simulink model "SerialComm"  (R2021a)
settings: Solver=FixedStepAuto  StartTime=0.0  StopTime=10.0  FixedStep=1e-3  RelTol=1e-3  EnableMultiTasking=on
undefined symbols (not defined in the file): A0, A1, D0, D1, D10, D11, D12, D13, D2, D3, D4, D5, D6, D7, D8, D9, magnitude, PTA0, PTA1, PTA2, PTB2, PTB23, PTB3, PTB9, PTC16, PTC17, PTC2, PTC3, PTC4, PTD0, PTD1, PTD2, PTD3
libraries: frdmk64flib x23, etargetslib x6, dspstat3 x1, simulink x1
(part 1 of 3)
settings Model: ExtModeTrigDuration=5  Creator=Arun Mistry  LastModifiedBy=Arun Mistry
settings OptimizationCC: EnhancedBackFolding=on  PassReuseOutputArgsAs=Individual arguments  ZeroExternalMemoryAtStartup=off  ZeroInternalMemoryAtStartup=off  MaxStackSize=64  OptimizeBlockOrder=speed  DifferentSizesBufferReuse=on  OptimizationCustomize=off  EfficientTunableParamExpr=on
settings DebuggingCC: ParameterTunabilityLossMsg=error
settings HardwareCC: ProdBitPerPointer=32  ProdBitPerSizeT=32  ProdBitPerPtrDiffT=32  ProdLargestAtomicInteger=Long  ProdLargestAtomicFloat=Double  ProdWordSize=32  ProdHWDeviceType=ARM Compatible->ARM Cortex
settings SFSimCC: MATLABDynamicMemAlloc=off
settings RTWCC: SystemTargetFile=ert.tlc  HardwareBoard=NXP FRDM-K64F  TLCOptions="-aInlineSetEventsForThisBaseRateFcn=TLC_FALSE -aSuppressMultiTaskScheduler=TLC_FALSE  -aRateBasedStepFcn=0"  TemplateMakefile=ert_default_tmf  Toolchain=GNU Tools for ARM Embedded Processors
settings CodeAppCC: ForceParamTrailComments=on  IgnoreCustomStorageClasses=off  OperatorAnnotations=on  SimulinkDataObjDesc=on  SFDataObjDesc=on  InsertBlockDesc=on
settings ERTTargetCC: ExtModeTransport=4  ExtModeMexFile=sendToCommService

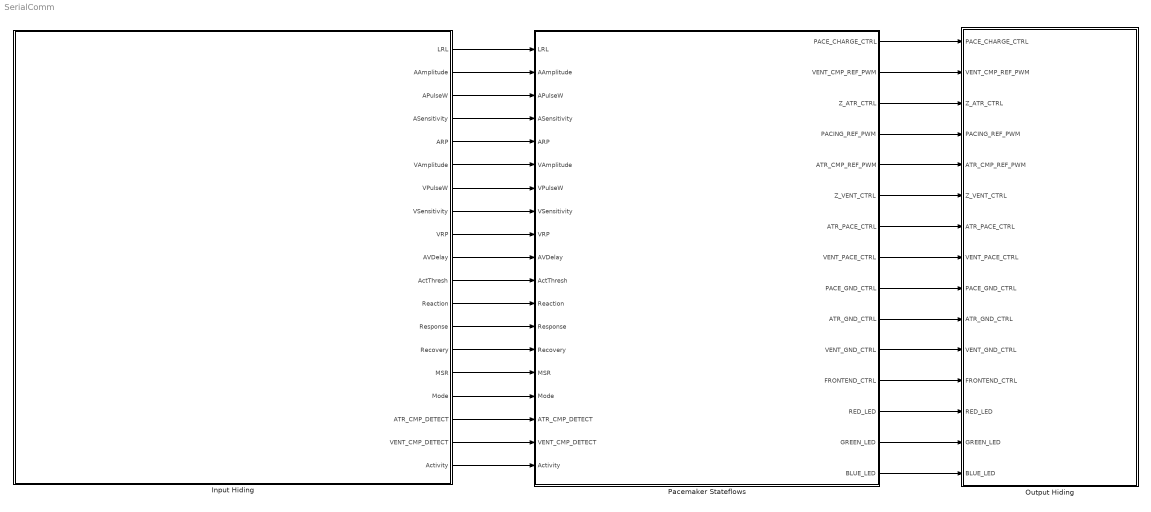
== system SerialComm ==
  Input Hiding : Subsystem
  Output Hiding : Subsystem
  Pacemaker Stateflows : Stateflow chart  TreatAsAtomicUnit=on
      settings: PortSchema="{\"entries\":[{\"content\":{\"sides\":[{\"content\":{\"connectorIds\":[\"In1\",\"In2\",\"In3\",\"In4\",\"In5\",\"In6\",\"In7\",\"In8\",\"In9\",\"In17\",\"In11\",\"In10\",\"In12\",\"In14\",\"In19\",\"In13\",\"In15\",\"In16\",\"In18\"]},\"type\":\"ConnectorPlacement.EquallySpacedRectSide\",\"uuid\":\"6f24296b-9994-4871-8227-e053a3629335\"},{\"content\":{\"connectorIds\":[\"Out1\",\"Out2\",\"Out3\",\"Out4\",\"Out5\",\"Out6\",\"Out7\",\"Out8\",\"Out9\",\"Out10\",\"Out11\",\"Out12\",\"Out13\",\"Out14\",\"Out15\"],\"side\":\"RIGHT\"},\"type\":\"ConnectorPlacement.EquallySpacedRectSide\",\"uuid\":\"36cf1f29-c3ea-48aa-b003-da737efff16a\"},{\"content\":{\"connectorIds\":[],\"side\":\"TOP\"},\"type\":\"ConnectorPlacement.EquallySpacedRectSide\",\"uuid\":\"8330eb51-0bc3-4d96-96ed-331fbb159cdb\"}]},\"type\":\"ConnectorPlacement.EquallySpacedConnector\",\"uuid\":\"1e79ed8a-065e-4a3c-97dd-23eb49490e0b\"}],\"packageUris\":[\"http://schema.mathworks.com/mf0/Connector/R2020b\"],\"version\":\"1.0\"}"
  wires:
  Input Hiding/14(Recovery) -> Pacemaker Stateflows/14(Recovery)
  Input Hiding/16(Mode) -> Pacemaker Stateflows/13(Mode)
  Pacemaker Stateflows/9(PACE_GND_CTRL) -> Output Hiding/9(PACE_GND_CTRL)
  Input Hiding/11(ActThresh) -> Pacemaker Stateflows/11(ActThresh)
  Input Hiding/9(VRP) -> Pacemaker Stateflows/9(VRP)
  Pacemaker Stateflows/5(ATR_CMP_REF_PWM) -> Output Hiding/5(ATR_CMP_REF_PWM)
  Input Hiding/8(VSensitivity) -> Pacemaker Stateflows/8(VSensitivity)
  Input Hiding/13(Response) -> Pacemaker Stateflows/12(Response)
  Input Hiding/19(Activity) -> Pacemaker Stateflows/18(Activity)
  Input Hiding/6(VAmplitude) -> Pacemaker Stateflows/6(VAmplitude)
  Pacemaker Stateflows/2(VENT_CMP_REF_PWM) -> Output Hiding/2(VENT_CMP_REF_PWM)
  Pacemaker Stateflows/8(VENT_PACE_CTRL) -> Output Hiding/8(VENT_PACE_CTRL)
  Pacemaker Stateflows/12(FRONTEND_CTRL) -> Output Hiding/12(FRONTEND_CTRL)
  Input Hiding/10(AVDelay) -> Pacemaker Stateflows/17(AVDelay)
  Pacemaker Stateflows/13(RED_LED) -> Output Hiding/13(RED_LED)
  Pacemaker Stateflows/3(Z_ATR_CTRL) -> Output Hiding/3(Z_ATR_CTRL)
  Pacemaker Stateflows/14(GREEN_LED) -> Output Hiding/14(GREEN_LED)
  Input Hiding/15(MSR) -> Pacemaker Stateflows/19(MSR)
  Input Hiding/4(ASensitivity) -> Pacemaker Stateflows/4(ASensitivity)
  Input Hiding/1(LRL) -> Pacemaker Stateflows/1(LRL)
  Input Hiding/5(ARP) -> Pacemaker Stateflows/5(ARP)
  Pacemaker Stateflows/11(VENT_GND_CTRL) -> Output Hiding/11(VENT_GND_CTRL)
  Input Hiding/12(Reaction) -> Pacemaker Stateflows/10(Reaction)
  Input Hiding/2(AAmplitude) -> Pacemaker Stateflows/2(AAmplitude)
  Pacemaker Stateflows/1(PACE_CHARGE_CTRL) -> Output Hiding/1(PACE_CHARGE_CTRL)
  Input Hiding/3(APulseW) -> Pacemaker Stateflows/3(APulseW)
  Pacemaker Stateflows/4(PACING_REF_PWM) -> Output Hiding/4(PACING_REF_PWM)
  Input Hiding/18(VENT_CMP_DETECT) -> Pacemaker Stateflows/16(VENT_CMP_DETECT)
  Input Hiding/17(ATR_CMP_DETECT) -> Pacemaker Stateflows/15(ATR_CMP_DETECT)
  Pacemaker Stateflows/7(ATR_PACE_CTRL) -> Output Hiding/7(ATR_PACE_CTRL)
  Input Hiding/7(VPulseW) -> Pacemaker Stateflows/7(VPulseW)
  Pacemaker Stateflows/10(ATR_GND_CTRL) -> Output Hiding/10(ATR_GND_CTRL)
  Pacemaker Stateflows/6(Z_VENT_CTRL) -> Output Hiding/6(Z_VENT_CTRL)
  Pacemaker Stateflows/15(BLUE_LED) -> Output Hiding/15(BLUE_LED)

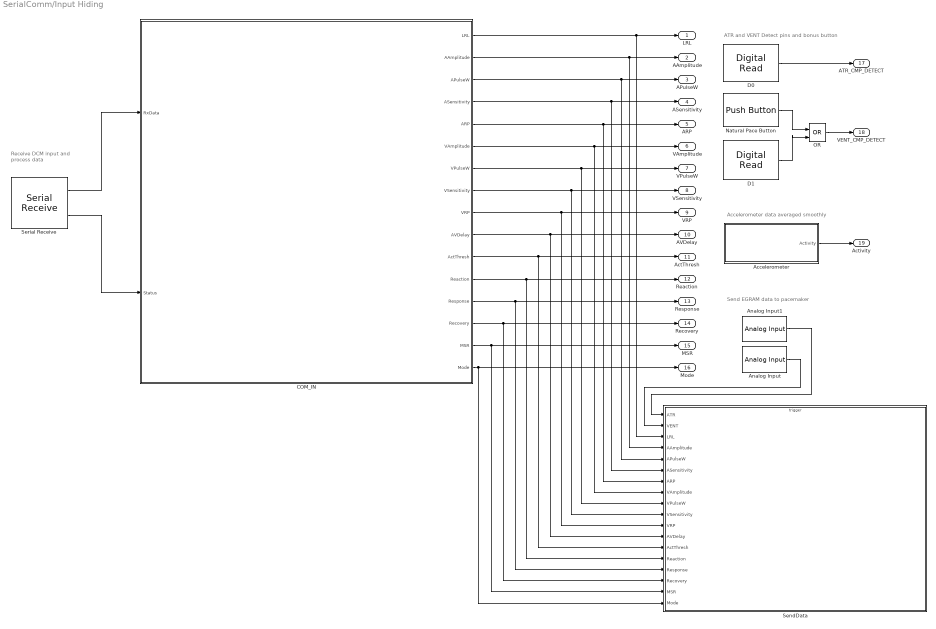
== system SerialComm/Input Hiding ==
  note: ATR and VENT Detect pins and bonus button
  note: Accelerometer data averaged smoothly
  note: Send EGRAM data to pacemaker
  note: Receive DCM input
      | and process data
  Accelerometer : Subsystem
  Analog Input : frdmk64flib/Analog Input  Whichpin=PTB3 (A1)  SampleTime=-1
  Analog Input1 : frdmk64flib/Analog Input  Whichpin=PTB2 (A0)  SampleTime=-1
  COM_IN : Stateflow chart  TreatAsAtomicUnit=on
  D0 : frdmk64flib/Digital Read  Whichpin=PTC16 (D0)  SampleTime=-1
  D1 : frdmk64flib/Digital Read  Whichpin=PTC17 (D1)  SampleTime=-1
  Natural Pace Button : frdmk64flib/Push Button  Whichswitch=SW3  SampleTime1=-1
  OR : Logic  Operator=OR  IconShape=distinctive  AllPortsSameDT=off  OutDataTypeStr=boolean
  SendData : Subsystem  TreatAsAtomicUnit=on
  Serial Receive : frdmk64flib/Serial Receive  SCIModule=0  Baudrate=uint32(9600)  Parity=None  StopBits=1  HardwareFlowControl=None  ByteOrder=LittleEndian  DataType=uint8  DataLength=22  BlockingMode=off  OutputStatus=on  SampleTime=-1
  LRL : Outport  OutDataTypeStr=uint16
  AAmplitude : Outport  Port=2  OutDataTypeStr=uint8
  APulseW : Outport  Port=3  OutDataTypeStr=uint8
  ASensitivity : Outport  Port=4  OutDataTypeStr=uint8
  ARP : Outport  Port=5  OutDataTypeStr=uint16
  VAmplitude : Outport  Port=6  OutDataTypeStr=uint8
  VPulseW : Outport  Port=7  OutDataTypeStr=uint8
  VSensitivity : Outport  Port=8  OutDataTypeStr=uint8
  VRP : Outport  Port=9  OutDataTypeStr=uint16
  AVDelay : Outport  Port=10  OutDataTypeStr=uint16
  ActThresh : Outport  Port=11  OutDataTypeStr=double
  Reaction : Outport  Port=12  OutDataTypeStr=uint8
  Response : Outport  Port=13  OutDataTypeStr=uint8
  Recovery : Outport  Port=14  OutDataTypeStr=uint16
  MSR : Outport  Port=15  OutDataTypeStr=uint16
  Mode : Outport  Port=16  OutDataTypeStr=uint8
  ATR_CMP_DETECT : Outport  Port=17  OutDataTypeStr=boolean
  VENT_CMP_DETECT : Outport  Port=18  OutDataTypeStr=boolean
  Activity : Outport  Port=19  OutDataTypeStr=double
  wires:
  COM_IN/3(APulseW) -> APulseW/1, SendData/5(APulseW)
  COM_IN/7(VPulseW) -> VPulseW/1, SendData/9(VPulseW)
  COM_IN/9(VRP) -> VRP/1, SendData/11(VRP)
  COM_IN/5(ARP) -> ARP/1, SendData/7(ARP)
  D0/1 -> ATR_CMP_DETECT/1
  COM_IN/1(LRL) -> LRL/1, SendData/3(LRL)
  COM_IN/10(AVDelay) -> AVDelay/1, SendData/12(AVDelay)
  COM_IN/6(VAmplitude) -> VAmplitude/1, SendData/8(VAmplitude)
  COM_IN/2(AAmplitude) -> AAmplitude/1, SendData/4(AAmplitude)
  Accelerometer/1(Activity) -> Activity/1
  COM_IN/12(Reaction) -> Reaction/1, SendData/14(Reaction)
  COM_IN/13(Response) -> Response/1, SendData/15(Response)
  COM_IN/14(Recovery) -> Recovery/1, SendData/16(Recovery)
  COM_IN/15(MSR) -> MSR/1, SendData/17(MSR)
  COM_IN/11(ActThresh) -> ActThresh/1, SendData/13(ActThresh)
  D1/1 -> OR/2
  OR/1 -> VENT_CMP_DETECT/1
  Natural Pace Button/1 -> OR/1
  COM_IN/4(ASensitivity) -> ASensitivity/1, SendData/6(ASensitivity)
  COM_IN/8(VSensitivity) -> VSensitivity/1, SendData/10(VSensitivity)
  Serial Receive/2 -> COM_IN/2(Status)
  Serial Receive/1 -> COM_IN/1(RxData)
  COM_IN/16(Mode) -> Mode/1, SendData/18(Mode)
  Analog Input/1 -> SendData/2(VENT)
  Analog Input1/1 -> SendData/1(ATR)

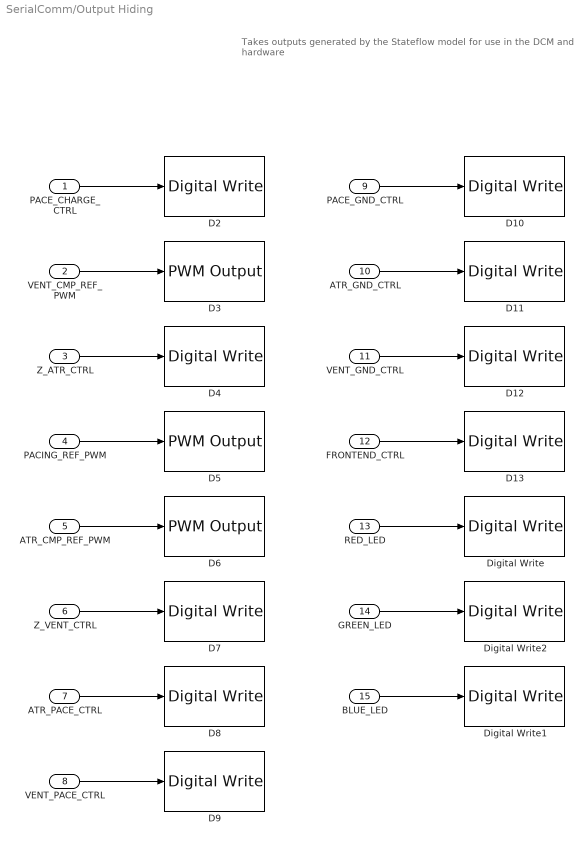
== system SerialComm/Output Hiding ==
  note: Takes outputs generated by the Stateflow model for use in the DCM and hardware
  PACE_CHARGE_CTRL : Inport  OutDataTypeStr=boolean
  VENT_CMP_REF_PWM : Inport  Port=2  OutDataTypeStr=uint8
  Z_ATR_CTRL : Inport  Port=3  OutDataTypeStr=boolean
  PACING_REF_PWM : Inport  Port=4  OutDataTypeStr=uint8
  ATR_CMP_REF_PWM : Inport  Port=5  OutDataTypeStr=uint8
  Z_VENT_CTRL : Inport  Port=6  OutDataTypeStr=boolean
  ATR_PACE_CTRL : Inport  Port=7  OutDataTypeStr=boolean
  VENT_PACE_CTRL : Inport  Port=8  OutDataTypeStr=boolean
  PACE_GND_CTRL : Inport  Port=9  OutDataTypeStr=boolean
  ATR_GND_CTRL : Inport  Port=10  OutDataTypeStr=boolean
  VENT_GND_CTRL : Inport  Port=11  OutDataTypeStr=boolean
  FRONTEND_CTRL : Inport  Port=12  OutDataTypeStr=boolean
  RED_LED : Inport  Port=13  OutDataTypeStr=boolean
  GREEN_LED : Inport  Port=14  OutDataTypeStr=boolean
  BLUE_LED : Inport  Port=15  OutDataTypeStr=boolean
  D10 : frdmk64flib/Digital Write  Whichpin=PTD0 (D10)
  D11 : frdmk64flib/Digital Write  Whichpin=PTD2 (D11)
  D12 : frdmk64flib/Digital Write  Whichpin=PTD3 (D12)
  D13 : frdmk64flib/Digital Write  Whichpin=PTD1 (D13)
  D2 : frdmk64flib/Digital Write  Whichpin=PTB9 (D2)
  D3 : frdmk64flib/PWM Output  Whichpin=PTA1 (D3)  InitialFrequency=2000  InitialDutyCycle=100
  D4 : frdmk64flib/Digital Write  Whichpin=PTB23 (D4)
  D5 : frdmk64flib/PWM Output  Whichpin=PTA2 (D5)  InitialFrequency=2000  InitialDutyCycle=100
  D6 : frdmk64flib/PWM Output  Whichpin=PTC2 (D6)  InitialFrequency=2000  InitialDutyCycle=100
  D7 : frdmk64flib/Digital Write  Whichpin=PTC3 (D7)
  "D8 " : frdmk64flib/Digital Write  Whichpin=PTA0 (D8)
  D9 : frdmk64flib/Digital Write  Whichpin=PTC4 (D9)
  Digital Write : frdmk64flib/Digital Write  Whichpin=RED_LED
  Digital Write1 : frdmk64flib/Digital Write  Whichpin=BLUE_LED
  Digital Write2 : frdmk64flib/Digital Write  Whichpin=GREEN_LED
  wires:
  VENT_PACE_CTRL/1 -> D9/1
  ATR_CMP_REF_PWM/1 -> D6/1
  PACE_GND_CTRL/1 -> D10/1
  VENT_CMP_REF_PWM/1 -> D3/1
  PACING_REF_PWM/1 -> D5/1
  ATR_GND_CTRL/1 -> D11/1
  ATR_PACE_CTRL/1 -> "D8 "/1
  PACE_CHARGE_CTRL/1 -> D2/1
  FRONTEND_CTRL/1 -> D13/1
  VENT_GND_CTRL/1 -> D12/1
  Z_ATR_CTRL/1 -> D4/1
  Z_VENT_CTRL/1 -> D7/1
  RED_LED/1 -> Digital Write/1
  BLUE_LED/1 -> Digital Write1/1
  GREEN_LED/1 -> Digital Write2/1

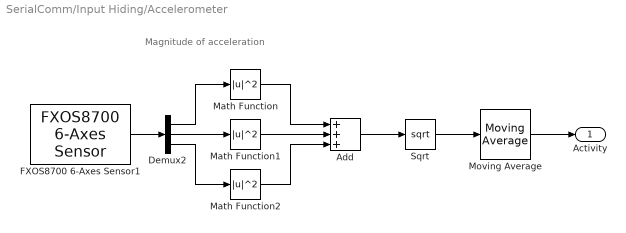
== system SerialComm/Input Hiding/Accelerometer ==
  note: Magnitude of acceleration
  Add : Sum  Inputs=+++
  Demux2 : Demux  Outputs=3
  FXOS8700 6-Axes Sensor1 : frdmk64flib/FXOS8700 6-Axes Sensor  Activesensor=Accelerometer only  ODR=100Hz  HybridODR=400Hz  Accelfullrange=-8g to +8g  SampleTime=1/100
  Math Function : Math  Operator=magnitude^2  SignedPower=on  OutDataTypeStr=double  SaturateOnIntegerOverflow=on
  Math Function1 : Math  Operator=magnitude^2  SignedPower=on  OutDataTypeStr=double  SaturateOnIntegerOverflow=on
  Math Function2 : Math  Operator=magnitude^2  SignedPower=on  OutDataTypeStr=double  SaturateOnIntegerOverflow=on
  Moving Average : dspstat3/Moving Average  Method=Sliding window  ForgettingFactorPort=off  SpecifyWindowLength=on  WindowLength=30  ForgettingFactor=0.9  SimulateUsing=Code generation
  Sqrt : Sqrt  SaturateOnIntegerOverflow=on
  Activity : Outport  OutDataTypeStr=double  SourceOfInitialOutputValue=Input signal
  wires:
  Sqrt/1 -> Moving Average/1
  FXOS8700 6-Axes Sensor1/1 -> Demux2/1
  Math Function/1 -> Add/1
  Add/1 -> Sqrt/1
  Math Function2/1 -> Add/3
  Demux2/2 -> Math Function1/1
  Math Function1/1 -> Add/2
  Demux2/1 -> Math Function/1
  Demux2/3 -> Math Function2/1
  Moving Average/1 -> Activity/1

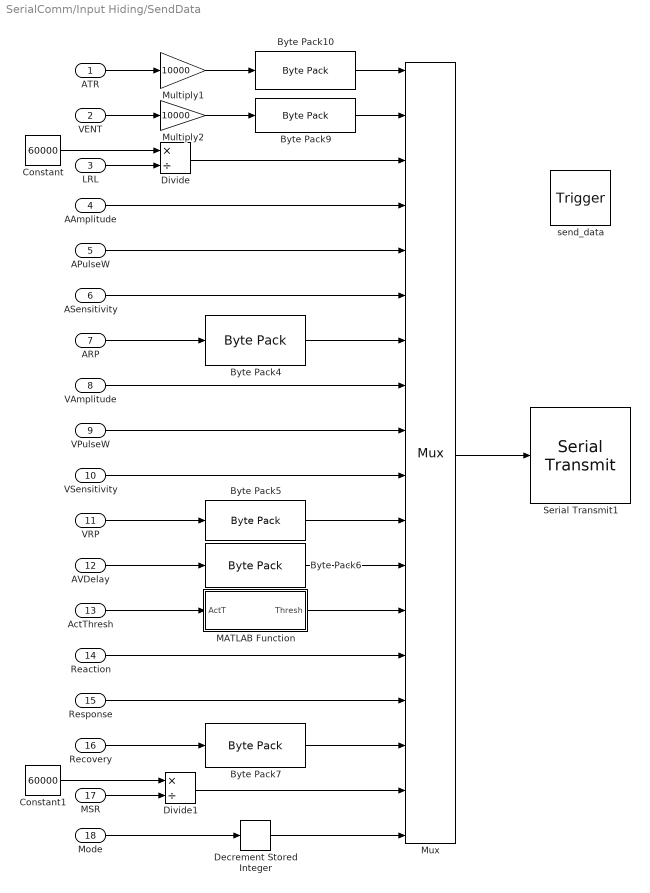
== system SerialComm/Input Hiding/SendData ==
  ATR : Inport
  VENT : Inport  Port=2
  LRL : Inport  Port=3
  AAmplitude : Inport  Port=4
  APulseW : Inport  Port=5
  ASensitivity : Inport  Port=6
  ARP : Inport  Port=7
  VAmplitude : Inport  Port=8
  VPulseW : Inport  Port=9
  VSensitivity : Inport  Port=10
  VRP : Inport  Port=11
  AVDelay : Inport  Port=12
  ActThresh : Inport  Port=13
  Reaction : Inport  Port=14
  Response : Inport  Port=15
  Recovery : Inport  Port=16
  MSR : Inport  Port=17
  Mode : Inport  Port=18
  send_data : TriggerPort  TriggerType=function-call  IsSimulinkFunction=on  FunctionName=send_data  VariantControl=Variant
  Byte Pack{4..7,9..10} (6 alike) : etargetslib/Byte Pack  datatypes={'uint16'}  byteAlign=1
  Constant : Constant  Value=60000
  Constant1 : Constant  Value=60000
  Decrement Stored Integer : simulink/Additional Math & Discrete/Additional Math: Increment - Decrement/Decrement Stored Integer
      settings: SourceProductBaseCode=SL
  Divide : Product  Inputs=*/  OutDataTypeStr=uint8
  Divide1 : Product  Inputs=*/  OutDataTypeStr=uint8
  MATLAB Function : MATLAB Function  TreatAsAtomicUnit=on
  Multiply1 : Gain  Gain=10000  OutDataTypeStr=uint16
  Multiply2 : Gain  Gain=10000  OutDataTypeStr=uint16
  Mux : Mux  Inputs=18
  Serial Transmit1 : frdmk64flib/Serial Transmit  SCIModule=0  Baudrate=uint32(9600)  Parity=None  StopBits=1  HardwareFlowControl=None  ByteOrder=LittleEndian  BlockingMode=on  OutputStatus=off
  wires:
  Mux/1 -> Serial Transmit1/1
  APulseW/1 -> Mux/5
  ASensitivity/1 -> Mux/6
  ARP/1 -> Byte Pack4/1
  VAmplitude/1 -> Mux/8
  VPulseW/1 -> Mux/9
  VSensitivity/1 -> Mux/10
  VRP/1 -> Byte Pack5/1
  AVDelay/1 -> Byte Pack6/1
  Reaction/1 -> Mux/14
  Response/1 -> Mux/15
  Recovery/1 -> Byte Pack7/1
  Mode/1 -> Decrement Stored Integer/1
  LRL/1 -> Divide/2
  Constant/1 -> Divide/1
  Constant1/1 -> Divide1/1
  MSR/1 -> Divide1/2
  Divide1/1 -> Mux/17
  Divide/1 -> Mux/3
  Byte Pack4/1 -> Mux/7
  Byte Pack5/1 -> Mux/11
  Byte Pack7/1 -> Mux/16
  Byte Pack6/1 -> Mux/12
  ATR/1 -> Multiply1/1
  VENT/1 -> Multiply2/1
  Byte Pack9/1 -> Mux/2
  Byte Pack10/1 -> Mux/1
  Multiply1/1 -> Byte Pack10/1
  Multiply2/1 -> Byte Pack9/1
  ActThresh/1 -> MATLAB Function/1(ActT)
  MATLAB Function/1(Thresh) -> Mux/13
  AAmplitude/1 -> Mux/4
  Decrement Stored Integer/1 -> Mux/18

== matlab function SerialComm/Input Hiding/SendData/MATLAB Function ==
  data: ActT input double; Thresh output uint8
function Thresh = fcn(ActT)
Thresh = uint8((ActT - 1)*2.5);
